simulink model "stereo_ibvs_core_backup_20260724_004703"  (R2025b)
settings: Solver=FixedStepDiscrete  StartTime=0.0  StopTime=inf  FixedStep=cfg.Ts  RelTol=1e-3
InitFcn:
  | cfgValid__=evalin('base','exist(''cfg'',''var'')==1 && isstruct(cfg) && all(isfield(cfg,{''Ts'',''robot'',''qInitial'',''zoomInitialSteps'',''cameraIntrinsicsStage1'',''rhoD'',''stereoBaseline'',''centerDesired'',''Kc'',''lambdaC'',''qMin'',''qMax'',''qLimitSoftMargin'',''qDotAlgorithmMax'',''stage1CalibrationReady''}))');if ~cfgValid__,modelFile__=get_param(bdroot,'FileName');modelDir__=fileparts(modelFile__);config1__=fullfile(modelDir__,'stereo_ibvs_config.m');config2__=fullfile(fileparts(modelDir__),'config','stereo_ibvs_config.m');if isfile(config1__),run(config1__);elseif isfile(config2__),run(config2__);else,error('StereoIBVS:ConfigNotFound','找不到stereo_ibvs_config.m。');end;end;clear cfgValid__ modelFile__ modelDir__ config1__ config2__
undefined symbols (not defined in the file): cfg, cfg_baseline, cfg_ekfCovarianceJitter, cfg_ekfInitializationMode, cfg_ekfP0, cfg_ekfRequireNewMeasurement, cfg_ekfSConditionMin, cfg_ekfX0, cfg_focalLength0Mm, cfg_fr3Axis, cfg_fr3Joint8OriginRPY, cfg_fr3Joint8OriginXYZ, cfg_fr3OriginRPY, cfg_fr3OriginXYZ, cfg_numericalEpsilon, cfg_pixelNoiseStd, cfg_q0, cfg_rhoMax, cfg_rhoMin, cfg_sigmaJerk, cfg_T_CL_CR, cfg_T_link8_CL, cfg_T_W_B, cfg_Ts, cfg_visibilityZMin
(part 1 of 4)
settings Model: Creator=harry  LastModifiedBy=harry

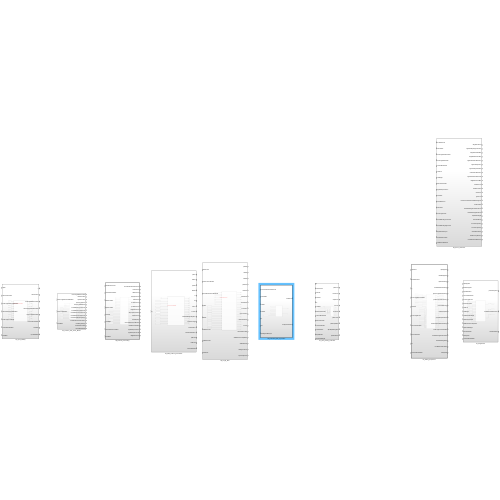
[thumbnail: Simulink's stored preview of the top-level diagram]
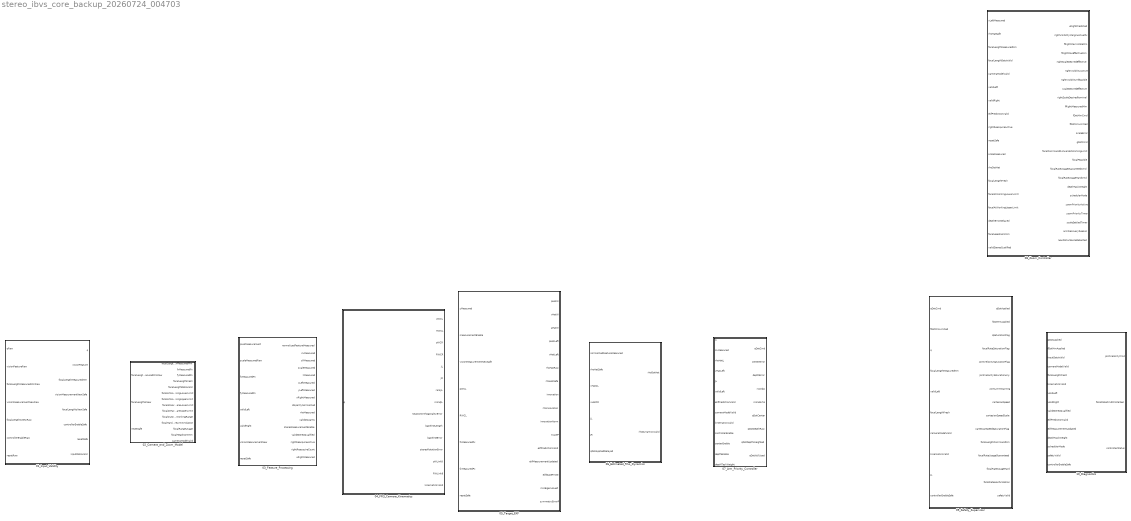
== system stereo_ibvs_core_backup_20260724_004703 ==
  01_Input_Validity : Subsystem
  02_Camera_and_Zoom_Model : Subsystem
  03_Feature_Processing : Subsystem  Description=将像素坐标转换为左右相机归一化坐标，并检查输入有效性。  TreatAsAtomicUnit=on
  04_FR3_Camera_Kinematics : Subsystem
  05_Target_EKF : Subsystem
  06_Estimated_Rho_Dynamics : Subsystem  TreatAsAtomicUnit=on
  07_Arm_Priority_Controller : Subsystem
  08_Zoom_Controller : Subsystem
  09_Safety_Supervisor : Subsystem  TreatAsAtomicUnit=on
  10_Diagnostics : Subsystem

== system stereo_ibvs_core_backup_20260724_004703/01_Input_Validity ==
  qRaw : Inport  OutDataTypeStr=double  PortDimensions=[7 1]
  visionFeatureRaw : Inport  Port=2  OutDataTypeStr=double  PortDimensions=[8 1]
  focalLengthMeasuredMmRaw : Inport  Port=3  OutDataTypeStr=double  PortDimensions=[2 1]
  visionMeasurementNewRaw : Inport  Port=4  OutDataTypeStr=double  PortDimensions=1
  focalLengthIsNewRaw : Inport  Port=5  OutDataTypeStr=double  PortDimensions=1
  controllerEnableRaw : Inport  Port=6  OutDataTypeStr=double  PortDimensions=1
  resetRaw : Inport  Port=7  OutDataTypeStr=double  PortDimensions=1
  Initial Focal Length Mm : Constant  Value=cfg_focalLength0Mm  OutDataTypeStr=double
  Initial Joint Position : Constant  Value=cfg_q0  OutDataTypeStr=double
  Input Validity : MATLAB Function  TreatAsAtomicUnit=on
  q : Outport  PortDimensions=[7 1]
  visionFeature : Outport  Port=2  PortDimensions=[8 1]
  focalLengthMeasuredMm : Outport  Port=3  PortDimensions=[2 1]
  visionMeasurementNewSafe : Outport  Port=4  PortDimensions=1
  focalLengthIsNewSafe : Outport  Port=5  PortDimensions=1
  controllerEnableSafe : Outport  Port=6  PortDimensions=1
  resetSafe : Outport  Port=7  PortDimensions=1
  inputDataValid : Outport  Port=8  PortDimensions=1
  wires:
  ? -> ?
  qRaw/1 -> Input Validity/1(qRaw)
  visionFeatureRaw/1 -> Input Validity/2(visionFeatureRaw)
  focalLengthMeasuredMmRaw/1 -> Input Validity/3(focalLengthMeasuredMmRaw)
  visionMeasurementNewRaw/1 -> Input Validity/4(visionMeasurementNewRaw)
  focalLengthIsNewRaw/1 -> Input Validity/5(focalLengthIsNewRaw)
  controllerEnableRaw/1 -> Input Validity/6(controllerEnableRaw)
  resetRaw/1 -> Input Validity/7(resetRaw)
  Initial Joint Position/1 -> Input Validity/8(qInitial)
  Initial Focal Length Mm/1 -> Input Validity/9(focalLength0Mm)
  Input Validity/1(q) -> q/1
  Input Validity/2(visionFeature) -> visionFeature/1
  Input Validity/3(focalLengthMeasuredMm) -> focalLengthMeasuredMm/1
  Input Validity/4(visionMeasurementNewSafe) -> visionMeasurementNewSafe/1
  Input Validity/5(focalLengthIsNewSafe) -> focalLengthIsNewSafe/1
  Input Validity/6(controllerEnableSafe) -> controllerEnableSafe/1
  Input Validity/7(resetSafe) -> resetSafe/1
  Input Validity/8(inputDataValid) -> inputDataValid/1

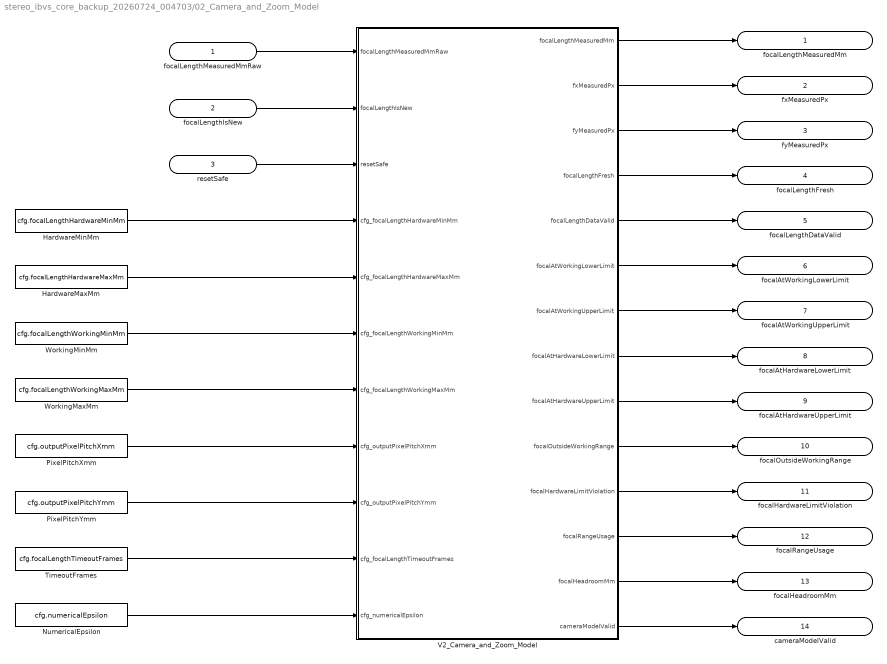
== system stereo_ibvs_core_backup_20260724_004703/02_Camera_and_Zoom_Model ==
  focalLengthMeasuredMmRaw : Inport  PortDimensions=2
  focalLengthIsNew : Inport  Port=2  PortDimensions=1
  resetSafe : Inport  Port=3  PortDimensions=1
  HardwareMaxMm : Constant  Value=cfg.focalLengthHardwareMaxMm
  HardwareMinMm : Constant  Value=cfg.focalLengthHardwareMinMm
  NumericalEpsilon : Constant  Value=cfg.numericalEpsilon
  PixelPitchXmm : Constant  Value=cfg.outputPixelPitchXmm
  PixelPitchYmm : Constant  Value=cfg.outputPixelPitchYmm
  TimeoutFrames : Constant  Value=cfg.focalLengthTimeoutFrames
  V2_Camera_and_Zoom_Model : MATLAB Function  TreatAsAtomicUnit=on
  WorkingMaxMm : Constant  Value=cfg.focalLengthWorkingMaxMm
  WorkingMinMm : Constant  Value=cfg.focalLengthWorkingMinMm
  focalLengthMeasuredMm : Outport  PortDimensions=2
  fxMeasuredPx : Outport  Port=2  PortDimensions=2
  fyMeasuredPx : Outport  Port=3  PortDimensions=2
  focalLengthFresh : Outport  Port=4  PortDimensions=1
  focalLengthDataValid : Outport  Port=5  PortDimensions=1
  focalAtWorkingLowerLimit : Outport  Port=6  PortDimensions=2
  focalAtWorkingUpperLimit : Outport  Port=7  PortDimensions=2
  focalAtHardwareLowerLimit : Outport  Port=8  PortDimensions=2
  focalAtHardwareUpperLimit : Outport  Port=9  PortDimensions=2
  focalOutsideWorkingRange : Outport  Port=10  PortDimensions=2
  focalHardwareLimitViolation : Outport  Port=11  PortDimensions=2
  focalRangeUsage : Outport  Port=12  PortDimensions=2
  focalHeadroomMm : Outport  Port=13  PortDimensions=2
  cameraModelValid : Outport  Port=14  PortDimensions=1
  wires:
  V2_Camera_and_Zoom_Model/13(focalHeadroomMm) -> focalHeadroomMm/1
  V2_Camera_and_Zoom_Model/12(focalRangeUsage) -> focalRangeUsage/1
  V2_Camera_and_Zoom_Model/11(focalHardwareLimitViolation) -> focalHardwareLimitViolation/1
  V2_Camera_and_Zoom_Model/10(focalOutsideWorkingRange) -> focalOutsideWorkingRange/1
  V2_Camera_and_Zoom_Model/14(cameraModelValid) -> cameraModelValid/1
  V2_Camera_and_Zoom_Model/9(focalAtHardwareUpperLimit) -> focalAtHardwareUpperLimit/1
  V2_Camera_and_Zoom_Model/6(focalAtWorkingLowerLimit) -> focalAtWorkingLowerLimit/1
  V2_Camera_and_Zoom_Model/4(focalLengthFresh) -> focalLengthFresh/1
  focalLengthMeasuredMmRaw/1 -> V2_Camera_and_Zoom_Model/1(focalLengthMeasuredMmRaw)
  focalLengthIsNew/1 -> V2_Camera_and_Zoom_Model/2(focalLengthIsNew)
  WorkingMinMm/1 -> V2_Camera_and_Zoom_Model/6(cfg_focalLengthWorkingMinMm)
  V2_Camera_and_Zoom_Model/3(fyMeasuredPx) -> fyMeasuredPx/1
  PixelPitchXmm/1 -> V2_Camera_and_Zoom_Model/8(cfg_outputPixelPitchXmm)
  V2_Camera_and_Zoom_Model/7(focalAtWorkingUpperLimit) -> focalAtWorkingUpperLimit/1
  TimeoutFrames/1 -> V2_Camera_and_Zoom_Model/10(cfg_focalLengthTimeoutFrames)
  V2_Camera_and_Zoom_Model/5(focalLengthDataValid) -> focalLengthDataValid/1
  resetSafe/1 -> V2_Camera_and_Zoom_Model/3(resetSafe)
  HardwareMinMm/1 -> V2_Camera_and_Zoom_Model/4(cfg_focalLengthHardwareMinMm)
  V2_Camera_and_Zoom_Model/8(focalAtHardwareLowerLimit) -> focalAtHardwareLowerLimit/1
  HardwareMaxMm/1 -> V2_Camera_and_Zoom_Model/5(cfg_focalLengthHardwareMaxMm)
  WorkingMaxMm/1 -> V2_Camera_and_Zoom_Model/7(cfg_focalLengthWorkingMaxMm)
  V2_Camera_and_Zoom_Model/1(focalLengthMeasuredMm) -> focalLengthMeasuredMm/1
  NumericalEpsilon/1 -> V2_Camera_and_Zoom_Model/11(cfg_numericalEpsilon)
  PixelPitchYmm/1 -> V2_Camera_and_Zoom_Model/9(cfg_outputPixelPitchYmm)
  V2_Camera_and_Zoom_Model/2(fxMeasuredPx) -> fxMeasuredPx/1

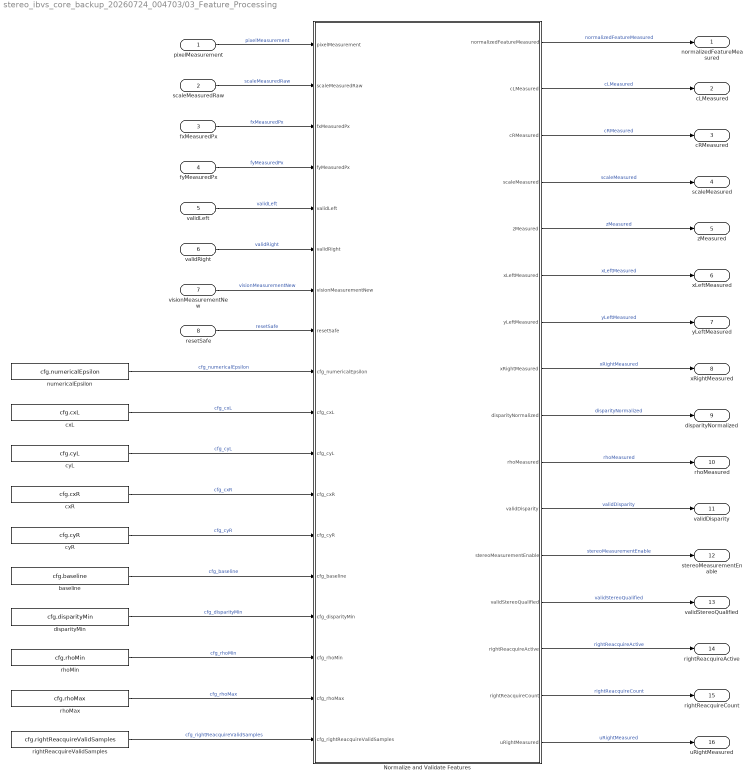
== system stereo_ibvs_core_backup_20260724_004703/03_Feature_Processing ==
  pixelMeasurement : Inport  OutDataTypeStr=double  PortDimensions=[4 1]
  scaleMeasuredRaw : Inport  Port=2  OutDataTypeStr=double  PortDimensions=[2 1]
  fxMeasuredPx : Inport  Port=3  OutDataTypeStr=double  PortDimensions=[2 1]
  fyMeasuredPx : Inport  Port=4  OutDataTypeStr=double  PortDimensions=[2 1]
  validLeft : Inport  Port=5  OutDataTypeStr=double  PortDimensions=1
  validRight : Inport  Port=6  OutDataTypeStr=double  PortDimensions=1
  visionMeasurementNew : Inport  Port=7  OutDataTypeStr=double  PortDimensions=1
  resetSafe : Inport  Port=8  OutDataTypeStr=double  PortDimensions=1
  Normalize and Validate Features : MATLAB Function  TreatAsAtomicUnit=on
  baseline : Constant  Value=cfg.baseline  OutDataTypeStr=double  SampleTime=-1
  cxL : Constant  Value=cfg.cxL  OutDataTypeStr=double  SampleTime=-1
  cxR : Constant  Value=cfg.cxR  OutDataTypeStr=double  SampleTime=-1
  cyL : Constant  Value=cfg.cyL  OutDataTypeStr=double  SampleTime=-1
  cyR : Constant  Value=cfg.cyR  OutDataTypeStr=double  SampleTime=-1
  disparityMin : Constant  Value=cfg.disparityMin  OutDataTypeStr=double  SampleTime=-1
  numericalEpsilon : Constant  Value=cfg.numericalEpsilon  OutDataTypeStr=double  SampleTime=-1
  rhoMax : Constant  Value=cfg.rhoMax  OutDataTypeStr=double  SampleTime=-1
  rhoMin : Constant  Value=cfg.rhoMin  OutDataTypeStr=double  SampleTime=-1
  rightReacquireValidSamples : Constant  Value=cfg.rightReacquireValidSamples  OutDataTypeStr=double  SampleTime=-1
  normalizedFeatureMeasured : Outport  PortDimensions=[4 1]
  cLMeasured : Outport  Port=2  PortDimensions=[2 1]
  cRMeasured : Outport  Port=3  PortDimensions=[2 1]
  scaleMeasured : Outport  Port=4  PortDimensions=[2 1]
  zMeasured : Outport  Port=5  PortDimensions=[3 1]
  xLeftMeasured : Outport  Port=6  PortDimensions=1
  yLeftMeasured : Outport  Port=7  PortDimensions=1
  xRightMeasured : Outport  Port=8  PortDimensions=1
  disparityNormalized : Outport  Port=9  PortDimensions=1
  rhoMeasured : Outport  Port=10  PortDimensions=1
  validDisparity : Outport  Port=11  PortDimensions=1
  stereoMeasurementEnable : Outport  Port=12  PortDimensions=1
  validStereoQualified : Outport  Port=13  PortDimensions=1
  rightReacquireActive : Outport  Port=14  PortDimensions=1
  rightReacquireCount : Outport  Port=15  PortDimensions=1
  uRightMeasured : Outport  Port=16  PortDimensions=1
  wires:
  pixelMeasurement/1 -> Normalize and Validate Features/1(pixelMeasurement)  "pixelMeasurement"
  scaleMeasuredRaw/1 -> Normalize and Validate Features/2(scaleMeasuredRaw)  "scaleMeasuredRaw"
  fxMeasuredPx/1 -> Normalize and Validate Features/3(fxMeasuredPx)  "fxMeasuredPx"
  fyMeasuredPx/1 -> Normalize and Validate Features/4(fyMeasuredPx)  "fyMeasuredPx"
  validLeft/1 -> Normalize and Validate Features/5(validLeft)  "validLeft"
  validRight/1 -> Normalize and Validate Features/6(validRight)  "validRight"
  visionMeasurementNew/1 -> Normalize and Validate Features/7(visionMeasurementNew)  "visionMeasurementNew"
  resetSafe/1 -> Normalize and Validate Features/8(resetSafe)  "resetSafe"
  numericalEpsilon/1 -> Normalize and Validate Features/9(cfg_numericalEpsilon)  "cfg_numericalEpsilon"
  cxL/1 -> Normalize and Validate Features/10(cfg_cxL)  "cfg_cxL"
  cyL/1 -> Normalize and Validate Features/11(cfg_cyL)  "cfg_cyL"
  cxR/1 -> Normalize and Validate Features/12(cfg_cxR)  "cfg_cxR"
  cyR/1 -> Normalize and Validate Features/13(cfg_cyR)  "cfg_cyR"
  baseline/1 -> Normalize and Validate Features/14(cfg_baseline)  "cfg_baseline"
  disparityMin/1 -> Normalize and Validate Features/15(cfg_disparityMin)  "cfg_disparityMin"
  rhoMin/1 -> Normalize and Validate Features/16(cfg_rhoMin)  "cfg_rhoMin"
  rhoMax/1 -> Normalize and Validate Features/17(cfg_rhoMax)  "cfg_rhoMax"
  rightReacquireValidSamples/1 -> Normalize and Validate Features/18(cfg_rightReacquireValidSamples)  "cfg_rightReacquireValidSamples"
  Normalize and Validate Features/1(normalizedFeatureMeasured) -> normalizedFeatureMeasured/1  "normalizedFeatureMeasured"
  Normalize and Validate Features/2(cLMeasured) -> cLMeasured/1  "cLMeasured"
  Normalize and Validate Features/3(cRMeasured) -> cRMeasured/1  "cRMeasured"
  Normalize and Validate Features/4(scaleMeasured) -> scaleMeasured/1  "scaleMeasured"
  Normalize and Validate Features/5(zMeasured) -> zMeasured/1  "zMeasured"
  Normalize and Validate Features/6(xLeftMeasured) -> xLeftMeasured/1  "xLeftMeasured"
  Normalize and Validate Features/7(yLeftMeasured) -> yLeftMeasured/1  "yLeftMeasured"
  Normalize and Validate Features/8(xRightMeasured) -> xRightMeasured/1  "xRightMeasured"
  Normalize and Validate Features/9(disparityNormalized) -> disparityNormalized/1  "disparityNormalized"
  Normalize and Validate Features/10(rhoMeasured) -> rhoMeasured/1  "rhoMeasured"
  Normalize and Validate Features/11(validDisparity) -> validDisparity/1  "validDisparity"
  Normalize and Validate Features/12(stereoMeasurementEnable) -> stereoMeasurementEnable/1  "stereoMeasurementEnable"
  Normalize and Validate Features/13(validStereoQualified) -> validStereoQualified/1  "validStereoQualified"
  Normalize and Validate Features/14(rightReacquireActive) -> rightReacquireActive/1  "rightReacquireActive"
  Normalize and Validate Features/15(rightReacquireCount) -> rightReacquireCount/1  "rightReacquireCount"
  Normalize and Validate Features/16(uRightMeasured) -> uRightMeasured/1  "uRightMeasured"

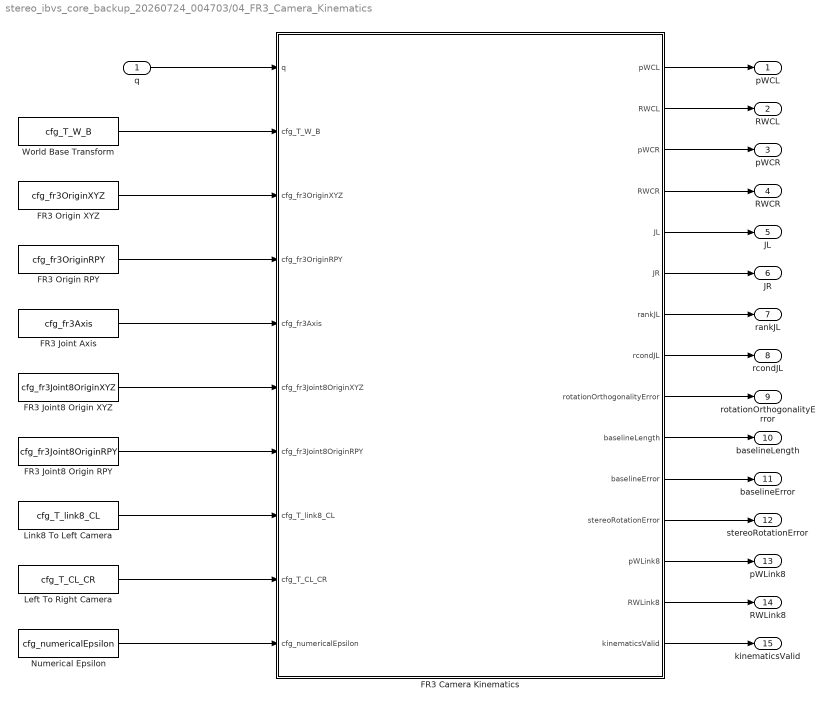
== system stereo_ibvs_core_backup_20260724_004703/04_FR3_Camera_Kinematics ==
  q : Inport  OutDataTypeStr=double  PortDimensions=[7 1]
  FR3 Camera Kinematics : MATLAB Function  TreatAsAtomicUnit=on
  FR3 Joint Axis : Constant  Value=cfg_fr3Axis  OutDataTypeStr=double  SampleTime=-1
  FR3 Joint8 Origin RPY : Constant  Value=cfg_fr3Joint8OriginRPY  OutDataTypeStr=double  SampleTime=-1
  FR3 Joint8 Origin XYZ : Constant  Value=cfg_fr3Joint8OriginXYZ  OutDataTypeStr=double  SampleTime=-1
  FR3 Origin RPY : Constant  Value=cfg_fr3OriginRPY  OutDataTypeStr=double  SampleTime=-1
  FR3 Origin XYZ : Constant  Value=cfg_fr3OriginXYZ  OutDataTypeStr=double  SampleTime=-1
  Left To Right Camera : Constant  Value=cfg_T_CL_CR  OutDataTypeStr=double  SampleTime=-1
  Link8 To Left Camera : Constant  Value=cfg_T_link8_CL  OutDataTypeStr=double  SampleTime=-1
  Numerical Epsilon : Constant  Value=cfg_numericalEpsilon  OutDataTypeStr=double  SampleTime=-1
  World Base Transform : Constant  Value=cfg_T_W_B  OutDataTypeStr=double  SampleTime=-1
  pWCL : Outport  PortDimensions=[3 1]
  RWCL : Outport  Port=2  PortDimensions=[3 3]
  pWCR : Outport  Port=3  PortDimensions=[3 1]
  RWCR : Outport  Port=4  PortDimensions=[3 3]
  JL : Outport  Port=5  PortDimensions=[6 7]
  JR : Outport  Port=6  PortDimensions=[6 7]
  rankJL : Outport  Port=7  PortDimensions=1
  rcondJL : Outport  Port=8  PortDimensions=1
  rotationOrthogonalityError : Outport  Port=9  PortDimensions=1
  baselineLength : Outport  Port=10  PortDimensions=1
  baselineError : Outport  Port=11  PortDimensions=1
  stereoRotationError : Outport  Port=12  PortDimensions=1
  pWLink8 : Outport  Port=13  PortDimensions=[3 1]
  RWLink8 : Outport  Port=14  PortDimensions=[3 3]
  kinematicsValid : Outport  Port=15  PortDimensions=1
  wires:
  ? -> ?
  q/1 -> FR3 Camera Kinematics/1(q)
  World Base Transform/1 -> FR3 Camera Kinematics/2(cfg_T_W_B)
  FR3 Origin XYZ/1 -> FR3 Camera Kinematics/3(cfg_fr3OriginXYZ)
  FR3 Origin RPY/1 -> FR3 Camera Kinematics/4(cfg_fr3OriginRPY)
  FR3 Joint Axis/1 -> FR3 Camera Kinematics/5(cfg_fr3Axis)
  FR3 Joint8 Origin XYZ/1 -> FR3 Camera Kinematics/6(cfg_fr3Joint8OriginXYZ)
  FR3 Joint8 Origin RPY/1 -> FR3 Camera Kinematics/7(cfg_fr3Joint8OriginRPY)
  Link8 To Left Camera/1 -> FR3 Camera Kinematics/8(cfg_T_link8_CL)
  Left To Right Camera/1 -> FR3 Camera Kinematics/9(cfg_T_CL_CR)
  Numerical Epsilon/1 -> FR3 Camera Kinematics/10(cfg_numericalEpsilon)
  FR3 Camera Kinematics/1(pWCL) -> pWCL/1
  FR3 Camera Kinematics/2(RWCL) -> RWCL/1
  FR3 Camera Kinematics/3(pWCR) -> pWCR/1
  FR3 Camera Kinematics/4(RWCR) -> RWCR/1
  FR3 Camera Kinematics/5(JL) -> JL/1
  FR3 Camera Kinematics/6(JR) -> JR/1
  FR3 Camera Kinematics/7(rankJL) -> rankJL/1
  FR3 Camera Kinematics/8(rcondJL) -> rcondJL/1
  FR3 Camera Kinematics/9(rotationOrthogonalityError) -> rotationOrthogonalityError/1
  FR3 Camera Kinematics/10(baselineLength) -> baselineLength/1
  FR3 Camera Kinematics/11(baselineError) -> baselineError/1
  FR3 Camera Kinematics/12(stereoRotationError) -> stereoRotationError/1
  FR3 Camera Kinematics/13(pWLink8) -> pWLink8/1
  FR3 Camera Kinematics/14(RWLink8) -> RWLink8/1
  FR3 Camera Kinematics/15(kinematicsValid) -> kinematicsValid/1

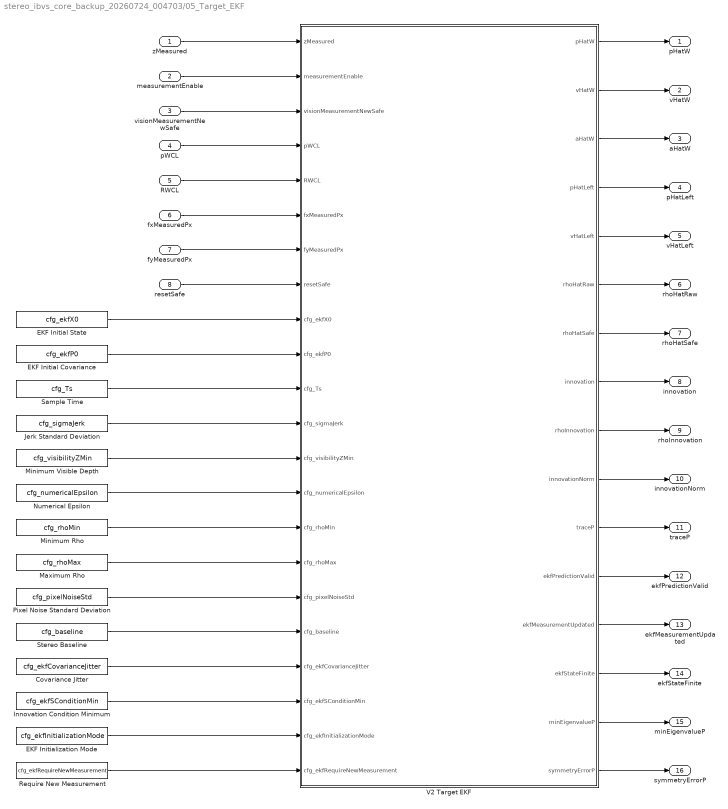
== system stereo_ibvs_core_backup_20260724_004703/05_Target_EKF ==
  zMeasured : Inport  OutDataTypeStr=double  PortDimensions=[3 1]
  measurementEnable : Inport  Port=2  OutDataTypeStr=double  PortDimensions=1
  visionMeasurementNewSafe : Inport  Port=3  OutDataTypeStr=double  PortDimensions=1
  pWCL : Inport  Port=4  OutDataTypeStr=double  PortDimensions=[3 1]
  RWCL : Inport  Port=5  OutDataTypeStr=double  PortDimensions=[3 3]
  fxMeasuredPx : Inport  Port=6  OutDataTypeStr=double  PortDimensions=[2 1]
  fyMeasuredPx : Inport  Port=7  OutDataTypeStr=double  PortDimensions=[2 1]
  resetSafe : Inport  Port=8  OutDataTypeStr=double  PortDimensions=1
  Covariance Jitter : Constant  Value=cfg_ekfCovarianceJitter  OutDataTypeStr=double  SampleTime=-1
  EKF Initial Covariance : Constant  Value=cfg_ekfP0  OutDataTypeStr=double  SampleTime=-1
  EKF Initial State : Constant  Value=cfg_ekfX0  OutDataTypeStr=double  SampleTime=-1
  EKF Initialization Mode : Constant  Value=cfg_ekfInitializationMode  OutDataTypeStr=double  SampleTime=-1
  Innovation Condition Minimum : Constant  Value=cfg_ekfSConditionMin  OutDataTypeStr=double  SampleTime=-1
  Jerk Standard Deviation : Constant  Value=cfg_sigmaJerk  OutDataTypeStr=double  SampleTime=-1
  Maximum Rho : Constant  Value=cfg_rhoMax  OutDataTypeStr=double  SampleTime=-1
  Minimum Rho : Constant  Value=cfg_rhoMin  OutDataTypeStr=double  SampleTime=-1
  Minimum Visible Depth : Constant  Value=cfg_visibilityZMin  OutDataTypeStr=double  SampleTime=-1
  Numerical Epsilon : Constant  Value=cfg_numericalEpsilon  OutDataTypeStr=double  SampleTime=-1
  Pixel Noise Standard Deviation : Constant  Value=cfg_pixelNoiseStd  OutDataTypeStr=double  SampleTime=-1
  Require New Measurement : Constant  Value=cfg_ekfRequireNewMeasurement  OutDataTypeStr=double  SampleTime=-1
  Sample Time : Constant  Value=cfg_Ts  OutDataTypeStr=double  SampleTime=-1
  Stereo Baseline : Constant  Value=cfg_baseline  OutDataTypeStr=double  SampleTime=-1
  V2 Target EKF : MATLAB Function  TreatAsAtomicUnit=on
  pHatW : Outport  PortDimensions=[3 1]
  vHatW : Outport  Port=2  PortDimensions=[3 1]
  aHatW : Outport  Port=3  PortDimensions=[3 1]
  pHatLeft : Outport  Port=4  PortDimensions=[3 1]
  vHatLeft : Outport  Port=5  PortDimensions=[3 1]
  rhoHatRaw : Outport  Port=6  PortDimensions=1
  rhoHatSafe : Outport  Port=7  PortDimensions=1
  innovation : Outport  Port=8  PortDimensions=[3 1]
  rhoInnovation : Outport  Port=9  PortDimensions=1
  innovationNorm : Outport  Port=10  PortDimensions=1
  traceP : Outport  Port=11  PortDimensions=1
  ekfPredictionValid : Outport  Port=12  PortDimensions=1
  ekfMeasurementUpdated : Outport  Port=13  PortDimensions=1
  ekfStateFinite : Outport  Port=14  PortDimensions=1
  minEigenvalueP : Outport  Port=15  PortDimensions=1
  symmetryErrorP : Outport  Port=16  PortDimensions=1
  wires:
  ? -> ?
  zMeasured/1 -> V2 Target EKF/1(zMeasured)
  measurementEnable/1 -> V2 Target EKF/2(measurementEnable)
  visionMeasurementNewSafe/1 -> V2 Target EKF/3(visionMeasurementNewSafe)
  pWCL/1 -> V2 Target EKF/4(pWCL)
  RWCL/1 -> V2 Target EKF/5(RWCL)
  fxMeasuredPx/1 -> V2 Target EKF/6(fxMeasuredPx)
  fyMeasuredPx/1 -> V2 Target EKF/7(fyMeasuredPx)
  resetSafe/1 -> V2 Target EKF/8(resetSafe)
  EKF Initial State/1 -> V2 Target EKF/9(cfg_ekfX0)
  EKF Initial Covariance/1 -> V2 Target EKF/10(cfg_ekfP0)
  Sample Time/1 -> V2 Target EKF/11(cfg_Ts)
  Jerk Standard Deviation/1 -> V2 Target EKF/12(cfg_sigmaJerk)
  Minimum Visible Depth/1 -> V2 Target EKF/13(cfg_visibilityZMin)
  Numerical Epsilon/1 -> V2 Target EKF/14(cfg_numericalEpsilon)
  Minimum Rho/1 -> V2 Target EKF/15(cfg_rhoMin)
  Maximum Rho/1 -> V2 Target EKF/16(cfg_rhoMax)
  Pixel Noise Standard Deviation/1 -> V2 Target EKF/17(cfg_pixelNoiseStd)
  Stereo Baseline/1 -> V2 Target EKF/18(cfg_baseline)
  Covariance Jitter/1 -> V2 Target EKF/19(cfg_ekfCovarianceJitter)
  Innovation Condition Minimum/1 -> V2 Target EKF/20(cfg_ekfSConditionMin)
  EKF Initialization Mode/1 -> V2 Target EKF/21(cfg_ekfInitializationMode)
  Require New Measurement/1 -> V2 Target EKF/22(cfg_ekfRequireNewMeasurement)
  V2 Target EKF/1(pHatW) -> pHatW/1
  V2 Target EKF/2(vHatW) -> vHatW/1
  V2 Target EKF/3(aHatW) -> aHatW/1
  V2 Target EKF/4(pHatLeft) -> pHatLeft/1
  V2 Target EKF/5(vHatLeft) -> vHatLeft/1
  V2 Target EKF/6(rhoHatRaw) -> rhoHatRaw/1
  V2 Target EKF/7(rhoHatSafe) -> rhoHatSafe/1
  V2 Target EKF/8(innovation) -> innovation/1
  V2 Target EKF/9(rhoInnovation) -> rhoInnovation/1
  V2 Target EKF/10(innovationNorm) -> innovationNorm/1
  V2 Target EKF/11(traceP) -> traceP/1
  V2 Target EKF/12(ekfPredictionValid) -> ekfPredictionValid/1
  V2 Target EKF/13(ekfMeasurementUpdated) -> ekfMeasurementUpdated/1
  V2 Target EKF/14(ekfStateFinite) -> ekfStateFinite/1
  V2 Target EKF/15(minEigenvalueP) -> minEigenvalueP/1
  V2 Target EKF/16(symmetryErrorP) -> symmetryErrorP/1

== system stereo_ibvs_core_backup_20260724_004703/06_Estimated_Rho_Dynamics ==
  normalizedFeatureMeasured : Inport  OutDataTypeStr=double  PortDimensions=[4 1]
  rhoHatSafe : Inport  Port=2  OutDataTypeStr=double  PortDimensions=1
  vHatCL : Inport  Port=3  OutDataTypeStr=double  PortDimensions=[3 1]
  vHatCR : Inport  Port=4  OutDataTypeStr=double  PortDimensions=[3 1]
  JL : Inport  Port=5  OutDataTypeStr=double  PortDimensions=[6 7]
  JR : Inport  Port=6  OutDataTypeStr=double  PortDimensions=[6 7]
  qDotAppliedDelayed : Inport  Port=7  OutDataTypeStr=double  PortDimensions=[7 1]
  Estimate Rho Dynamics : MATLAB Function  TreatAsAtomicUnit=on
  numericalEpsilon : Constant  Value=cfg.numericalEpsilon  OutDataTypeStr=double  SampleTime=-1
  rhoDotHat : Outport  PortDimensions=[2 1]
  rhoDynamicsValid : Outport  Port=2  PortDimensions=1
  wires:
  normalizedFeatureMeasured/1 -> Estimate Rho Dynamics/1(normalizedFeatureMeasured)  "normalizedFeatureMeasured"
  rhoHatSafe/1 -> Estimate Rho Dynamics/2(rhoHatSafe)  "rhoHatSafe"
  vHatCL/1 -> Estimate Rho Dynamics/3(vHatCL)  "vHatCL"
  vHatCR/1 -> Estimate Rho Dynamics/4(vHatCR)  "vHatCR"
  JL/1 -> Estimate Rho Dynamics/5(JL)  "JL"
  JR/1 -> Estimate Rho Dynamics/6(JR)  "JR"
  qDotAppliedDelayed/1 -> Estimate Rho Dynamics/7(qDotAppliedDelayed)  "qDotAppliedDelayed"
  numericalEpsilon/1 -> Estimate Rho Dynamics/8(cfg_numericalEpsilon)  "cfg_numericalEpsilon"
  Estimate Rho Dynamics/1(rhoDotHat) -> rhoDotHat/1  "rhoDotHat"
  Estimate Rho Dynamics/2(rhoDynamicsValid) -> rhoDynamicsValid/1  "rhoDynamicsValid"

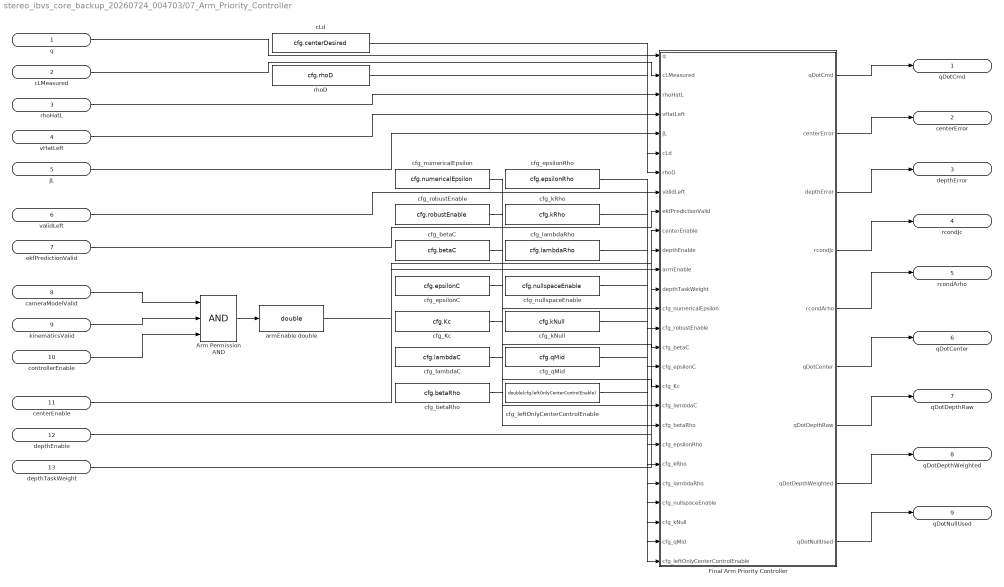
== system stereo_ibvs_core_backup_20260724_004703/07_Arm_Priority_Controller ==
  q : Inport
  cLMeasured : Inport  Port=2
  rhoHatL : Inport  Port=3
  vHatLeft : Inport  Port=4
  JL : Inport  Port=5
  validLeft : Inport  Port=6
  ekfPredictionValid : Inport  Port=7
  cameraModelValid : Inport  Port=8
  kinematicsValid : Inport  Port=9
  controllerEnable : Inport  Port=10
  centerEnable : Inport  Port=11
  depthEnable : Inport  Port=12
  depthTaskWeight : Inport  Port=13
  Arm Permission AND : Logic  Inputs=3  AllPortsSameDT=off  OutDataTypeStr=boolean
  Final Arm Priority Controller : MATLAB Function  TreatAsAtomicUnit=on
  armEnable double : DataTypeConversion  OutDataTypeStr=double  SaturateOnIntegerOverflow=off  RndMeth=Floor
  cLd : Constant  Value=cfg.centerDesired  OutDataTypeStr=double
  cfg_Kc : Constant  Value=cfg.Kc  OutDataTypeStr=double
  cfg_betaC : Constant  Value=cfg.betaC  OutDataTypeStr=double
  cfg_betaRho : Constant  Value=cfg.betaRho  OutDataTypeStr=double
  cfg_epsilonC : Constant  Value=cfg.epsilonC  OutDataTypeStr=double
  cfg_epsilonRho : Constant  Value=cfg.epsilonRho  OutDataTypeStr=double
  cfg_kNull : Constant  Value=cfg.kNull  OutDataTypeStr=double
  cfg_kRho : Constant  Value=cfg.kRho  OutDataTypeStr=double
  cfg_lambdaC : Constant  Value=cfg.lambdaC  OutDataTypeStr=double
  cfg_lambdaRho : Constant  Value=cfg.lambdaRho  OutDataTypeStr=double
  cfg_leftOnlyCenterControlEnable : Constant  Value=double(cfg.leftOnlyCenterControlEnable)  OutDataTypeStr=double
  cfg_nullspaceEnable : Constant  Value=cfg.nullspaceEnable  OutDataTypeStr=double
  cfg_numericalEpsilon : Constant  Value=cfg.numericalEpsilon  OutDataTypeStr=double
  cfg_qMid : Constant  Value=cfg.qMid  OutDataTypeStr=double
  cfg_robustEnable : Constant  Value=cfg.robustEnable  OutDataTypeStr=double
  rhoD : Constant  Value=cfg.rhoD  OutDataTypeStr=double
  qDotCmd : Outport
  centerError : Outport  Port=2
  depthError : Outport  Port=3
  rcondJc : Outport  Port=4
  rcondArho : Outport  Port=5
  qDotCenter : Outport  Port=6
  qDotDepthRaw : Outport  Port=7
  qDotDepthWeighted : Outport  Port=8
  qDotNullUsed : Outport  Port=9
  wires:
  cameraModelValid/1 -> Arm Permission AND/1
  kinematicsValid/1 -> Arm Permission AND/2
  controllerEnable/1 -> Arm Permission AND/3
  Arm Permission AND/1 -> armEnable double/1
  q/1 -> Final Arm Priority Controller/1(q)
  cLMeasured/1 -> Final Arm Priority Controller/2(cLMeasured)
  rhoHatL/1 -> Final Arm Priority Controller/3(rhoHatL)
  vHatLeft/1 -> Final Arm Priority Controller/4(vHatLeft)
  JL/1 -> Final Arm Priority Controller/5(JL)
  cLd/1 -> Final Arm Priority Controller/6(cLd)
  rhoD/1 -> Final Arm Priority Controller/7(rhoD)
  validLeft/1 -> Final Arm Priority Controller/8(validLeft)
  ekfPredictionValid/1 -> Final Arm Priority Controller/9(ekfPredictionValid)
  centerEnable/1 -> Final Arm Priority Controller/10(centerEnable)
  depthEnable/1 -> Final Arm Priority Controller/11(depthEnable)
  armEnable double/1 -> Final Arm Priority Controller/12(armEnable)
  depthTaskWeight/1 -> Final Arm Priority Controller/13(depthTaskWeight)
  cfg_numericalEpsilon/1 -> Final Arm Priority Controller/14(cfg_numericalEpsilon)
  cfg_robustEnable/1 -> Final Arm Priority Controller/15(cfg_robustEnable)
  cfg_betaC/1 -> Final Arm Priority Controller/16(cfg_betaC)
  cfg_epsilonC/1 -> Final Arm Priority Controller/17(cfg_epsilonC)
  cfg_Kc/1 -> Final Arm Priority Controller/18(cfg_Kc)
  cfg_lambdaC/1 -> Final Arm Priority Controller/19(cfg_lambdaC)
  cfg_betaRho/1 -> Final Arm Priority Controller/20(cfg_betaRho)
  cfg_epsilonRho/1 -> Final Arm Priority Controller/21(cfg_epsilonRho)
  cfg_kRho/1 -> Final Arm Priority Controller/22(cfg_kRho)
  cfg_lambdaRho/1 -> Final Arm Priority Controller/23(cfg_lambdaRho)
  cfg_nullspaceEnable/1 -> Final Arm Priority Controller/24(cfg_nullspaceEnable)
  cfg_kNull/1 -> Final Arm Priority Controller/25(cfg_kNull)
  cfg_qMid/1 -> Final Arm Priority Controller/26(cfg_qMid)
  cfg_leftOnlyCenterControlEnable/1 -> Final Arm Priority Controller/27(cfg_leftOnlyCenterControlEnable)
  Final Arm Priority Controller/1(qDotCmd) -> qDotCmd/1
  Final Arm Priority Controller/2(centerError) -> centerError/1
  Final Arm Priority Controller/3(depthError) -> depthError/1
  Final Arm Priority Controller/4(rcondJc) -> rcondJc/1
  Final Arm Priority Controller/5(rcondArho) -> rcondArho/1
  Final Arm Priority Controller/6(qDotCenter) -> qDotCenter/1
  Final Arm Priority Controller/7(qDotDepthRaw) -> qDotDepthRaw/1
  Final Arm Priority Controller/8(qDotDepthWeighted) -> qDotDepthWeighted/1
  Final Arm Priority Controller/9(qDotNullUsed) -> qDotNullUsed/1

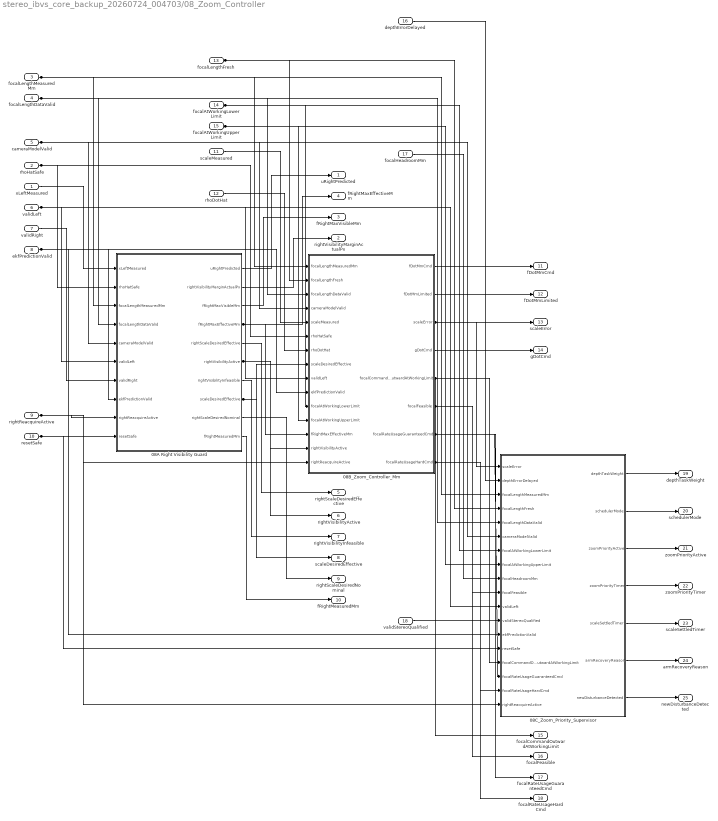
== system stereo_ibvs_core_backup_20260724_004703/08_Zoom_Controller ==
  xLeftMeasured : Inport  OutDataTypeStr=double  PortDimensions=1
  rhoHatSafe : Inport  Port=2  OutDataTypeStr=double  PortDimensions=1
  focalLengthMeasuredMm : Inport  Port=3  OutDataTypeStr=double  PortDimensions=[2 1]
  focalLengthDataValid : Inport  Port=4  OutDataTypeStr=double  PortDimensions=1
  cameraModelValid : Inport  Port=5  OutDataTypeStr=double  PortDimensions=1
  validLeft : Inport  Port=6  OutDataTypeStr=double  PortDimensions=1
  validRight : Inport  Port=7  OutDataTypeStr=double  PortDimensions=1
  ekfPredictionValid : Inport  Port=8  OutDataTypeStr=double  PortDimensions=1
  rightReacquireActive : Inport  Port=9  OutDataTypeStr=double  PortDimensions=1
  resetSafe : Inport  Port=10  OutDataTypeStr=double  PortDimensions=1
  scaleMeasured : Inport  Port=11  OutDataTypeStr=double  PortDimensions=[2 1]
  rhoDotHat : Inport  Port=12  OutDataTypeStr=double  PortDimensions=[2 1]
  focalLengthFresh : Inport  Port=13  OutDataTypeStr=double  PortDimensions=1
  focalAtWorkingLowerLimit : Inport  Port=14  OutDataTypeStr=double  PortDimensions=[2 1]
  focalAtWorkingUpperLimit : Inport  Port=15  OutDataTypeStr=double  PortDimensions=[2 1]
  depthErrorDelayed : Inport  Port=16  OutDataTypeStr=double  PortDimensions=1
  focalHeadroomMm : Inport  Port=17  OutDataTypeStr=double  PortDimensions=[2 1]
  validStereoQualified : Inport  Port=18  OutDataTypeStr=double  PortDimensions=1
  08A Right Visibility Guard : Subsystem
  08B_Zoom_Controller_Mm : Subsystem
  08C_Zoom_Priority_Supervisor : Subsystem
  uRightPredicted : Outport  PortDimensions=1
  rightVisibilityMarginActualPx : Outport  Port=2  PortDimensions=1
  fRightMaxVisibleMm : Outport  Port=3  PortDimensions=1
  fRightMaxEffectiveMm : Outport  Port=4  PortDimensions=1
  rightScaleDesiredEffective : Outport  Port=5  PortDimensions=1
  rightVisibilityActive : Outport  Port=6  PortDimensions=1
  rightVisibilityInfeasible : Outport  Port=7  PortDimensions=1
  scaleDesiredEffective : Outport  Port=8  PortDimensions=[2 1]
  rightScaleDesiredNominal : Outport  Port=9  PortDimensions=1
  fRightMeasuredMm : Outport  Port=10  PortDimensions=1
  fDotMmCmd : Outport  Port=11  PortDimensions=[2 1]
  fDotMmLimited : Outport  Port=12  PortDimensions=[2 1]
  scaleError : Outport  Port=13  PortDimensions=[2 1]
  gDotCmd : Outport  Port=14  PortDimensions=[2 1]
  focalCommandOutwardAtWorkingLimit : Outport  Port=15  PortDimensions=[2 1]
  focalFeasible : Outport  Port=16  PortDimensions=[2 1]
  focalRateUsageGuaranteedCmd : Outport  Port=17  PortDimensions=[2 1]
  focalRateUsageHardCmd : Outport  Port=18  PortDimensions=[2 1]
  depthTaskWeight : Outport  Port=19  PortDimensions=1
  schedulerMode : Outport  Port=20  PortDimensions=1
  zoomPriorityActive : Outport  Port=21  PortDimensions=1
  zoomPriorityTimer : Outport  Port=22  PortDimensions=1
  scaleSettledTimer : Outport  Port=23  PortDimensions=1
  armRecoveryReason : Outport  Port=24  PortDimensions=1
  newDisturbanceDetected : Outport  Port=25  PortDimensions=1
  wires:
  08C_Zoom_Priority_Supervisor/6(armRecoveryReason) -> armRecoveryReason/1
  08C_Zoom_Priority_Supervisor/5(scaleSettledTimer) -> scaleSettledTimer/1
  08C_Zoom_Priority_Supervisor/4(zoomPriorityTimer) -> zoomPriorityTimer/1
  08C_Zoom_Priority_Supervisor/2(schedulerMode) -> schedulerMode/1
  08C_Zoom_Priority_Supervisor/1(depthTaskWeight) -> depthTaskWeight/1
  08B_Zoom_Controller_Mm/8(focalRateUsageHardCmd) -> focalRateUsageHardCmd/1, 08C_Zoom_Priority_Supervisor/17(focalRateUsageHardCmd)
  08B_Zoom_Controller_Mm/5(focalCommandOutwardAtWorkingLimit) -> focalCommandOutwardAtWorkingLimit/1, 08C_Zoom_Priority_Supervisor/15(focalCommandOutwardAtWorkingLimit)
  08C_Zoom_Priority_Supervisor/7(newDisturbanceDetected) -> newDisturbanceDetected/1
  08B_Zoom_Controller_Mm/4(gDotCmd) -> gDotCmd/1
  08B_Zoom_Controller_Mm/3(scaleError) -> scaleError/1, 08C_Zoom_Priority_Supervisor/1(scaleError)
  focalAtWorkingLowerLimit/1 -> 08B_Zoom_Controller_Mm/11(focalAtWorkingLowerLimit), 08C_Zoom_Priority_Supervisor/7(focalAtWorkingLowerLimit)
  ekfPredictionValid/1 -> 08A Right Visibility Guard/8(ekfPredictionValid), 08B_Zoom_Controller_Mm/10(ekfPredictionValid), 08C_Zoom_Priority_Supervisor/13(ekfPredictionValid)
  08A Right Visibility Guard/7(rightVisibilityInfeasible) -> rightVisibilityInfeasible/1
  validRight/1 -> 08A Right Visibility Guard/7(validRight)
  validStereoQualified/1 -> 08C_Zoom_Priority_Supervisor/12(validStereoQualified)
  depthErrorDelayed/1 -> 08C_Zoom_Priority_Supervisor/2(depthErrorDelayed)
  08A Right Visibility Guard/3(fRightMaxVisibleMm) -> fRightMaxVisibleMm/1
  rightReacquireActive/1 -> 08A Right Visibility Guard/9(rightReacquireActive), 08B_Zoom_Controller_Mm/15(rightReacquireActive), 08C_Zoom_Priority_Supervisor/18(rightReacquireActive)
  rhoHatSafe/1 -> 08A Right Visibility Guard/2(rhoHatSafe), 08B_Zoom_Controller_Mm/6(rhoHatSafe)
  resetSafe/1 -> 08A Right Visibility Guard/10(resetSafe), 08C_Zoom_Priority_Supervisor/14(resetSafe)
  validLeft/1 -> 08A Right Visibility Guard/6(validLeft), 08C_Zoom_Priority_Supervisor/11(validLeft), 08B_Zoom_Controller_Mm/9(validLeft)
  cameraModelValid/1 -> 08A Right Visibility Guard/5(cameraModelValid), 08B_Zoom_Controller_Mm/4(cameraModelValid), 08C_Zoom_Priority_Supervisor/6(cameraModelValid)
  focalLengthDataValid/1 -> 08A Right Visibility Guard/4(focalLengthDataValid), 08B_Zoom_Controller_Mm/3(focalLengthDataValid), 08C_Zoom_Priority_Supervisor/5(focalLengthDataValid)
  08A Right Visibility Guard/1(uRightPredicted) -> uRightPredicted/1
  focalLengthFresh/1 -> 08B_Zoom_Controller_Mm/2(focalLengthFresh), 08C_Zoom_Priority_Supervisor/4(focalLengthFresh)
  focalLengthMeasuredMm/1 -> 08A Right Visibility Guard/3(focalLengthMeasuredMm), 08B_Zoom_Controller_Mm/1(focalLengthMeasuredMm), 08C_Zoom_Priority_Supervisor/3(focalLengthMeasuredMm)
  08B_Zoom_Controller_Mm/6(focalFeasible) -> focalFeasible/1, 08C_Zoom_Priority_Supervisor/10(focalFeasible)
  scaleMeasured/1 -> 08B_Zoom_Controller_Mm/5(scaleMeasured)
  08A Right Visibility Guard/9(rightScaleDesiredNominal) -> rightScaleDesiredNominal/1
  rhoDotHat/1 -> 08B_Zoom_Controller_Mm/7(rhoDotHat)
  xLeftMeasured/1 -> 08A Right Visibility Guard/1(xLeftMeasured)
  08A Right Visibility Guard/2(rightVisibilityMarginActualPx) -> rightVisibilityMarginActualPx/1
  08B_Zoom_Controller_Mm/7(focalRateUsageGuaranteedCmd) -> focalRateUsageGuaranteedCmd/1, 08C_Zoom_Priority_Supervisor/16(focalRateUsageGuaranteedCmd)
  08A Right Visibility Guard/4(fRightMaxEffectiveMm) -> fRightMaxEffectiveMm/1, 08B_Zoom_Controller_Mm/13(fRightMaxEffectiveMm)
  08A Right Visibility Guard/8(scaleDesiredEffective) -> scaleDesiredEffective/1, 08B_Zoom_Controller_Mm/8(scaleDesiredEffective)
  focalAtWorkingUpperLimit/1 -> 08B_Zoom_Controller_Mm/12(focalAtWorkingUpperLimit), 08C_Zoom_Priority_Supervisor/8(focalAtWorkingUpperLimit)
  08A Right Visibility Guard/6(rightVisibilityActive) -> rightVisibilityActive/1, 08B_Zoom_Controller_Mm/14(rightVisibilityActive)
  focalHeadroomMm/1 -> 08C_Zoom_Priority_Supervisor/9(focalHeadroomMm)
  08A Right Visibility Guard/10(fRightMeasuredMm) -> fRightMeasuredMm/1
  08A Right Visibility Guard/5(rightScaleDesiredEffective) -> rightScaleDesiredEffective/1
  08B_Zoom_Controller_Mm/1(fDotMmCmd) -> fDotMmCmd/1
  08C_Zoom_Priority_Supervisor/3(zoomPriorityActive) -> zoomPriorityActive/1
  08B_Zoom_Controller_Mm/2(fDotMmLimited) -> fDotMmLimited/1

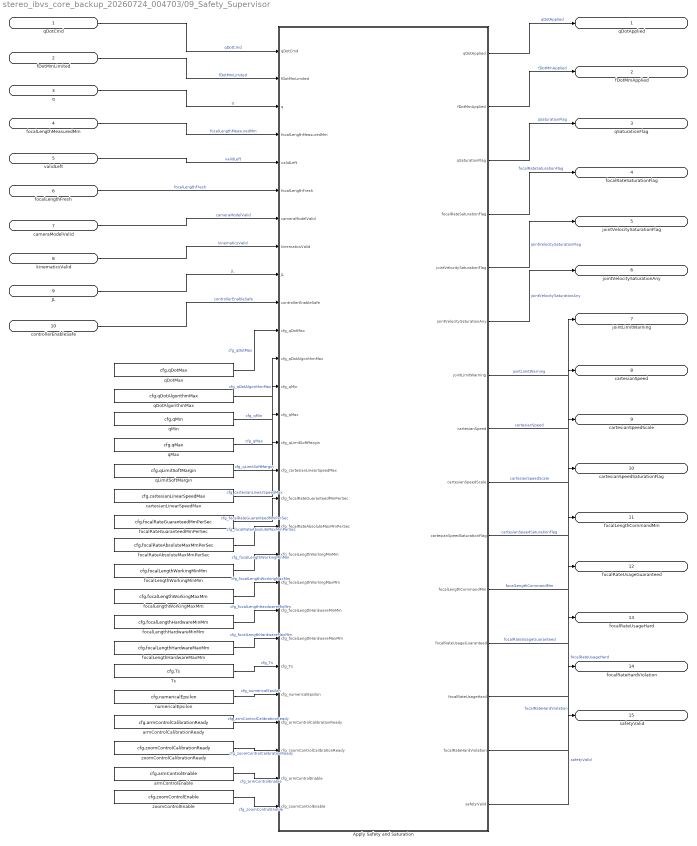
== system stereo_ibvs_core_backup_20260724_004703/09_Safety_Supervisor ==
  qDotCmd : Inport  OutDataTypeStr=double  PortDimensions=[7 1]
  fDotMmLimited : Inport  Port=2  OutDataTypeStr=double  PortDimensions=[2 1]
  q : Inport  Port=3  OutDataTypeStr=double  PortDimensions=[7 1]
  focalLengthMeasuredMm : Inport  Port=4  OutDataTypeStr=double  PortDimensions=[2 1]
  validLeft : Inport  Port=5  OutDataTypeStr=double  PortDimensions=1
  focalLengthFresh : Inport  Port=6  OutDataTypeStr=double  PortDimensions=1
  cameraModelValid : Inport  Port=7  OutDataTypeStr=double  PortDimensions=1
  kinematicsValid : Inport  Port=8  OutDataTypeStr=double  PortDimensions=1
  JL : Inport  Port=9  OutDataTypeStr=double  PortDimensions=[6 7]
  controllerEnableSafe : Inport  Port=10  OutDataTypeStr=double  PortDimensions=1
  Apply Safety and Saturation : MATLAB Function  TreatAsAtomicUnit=on
  Ts : Constant  Value=cfg.Ts  OutDataTypeStr=double  SampleTime=-1
  armControlCalibrationReady : Constant  Value=cfg.armControlCalibrationReady  OutDataTypeStr=double  SampleTime=-1
  armControlEnable : Constant  Value=cfg.armControlEnable  OutDataTypeStr=double  SampleTime=-1
  cartesianLinearSpeedMax : Constant  Value=cfg.cartesianLinearSpeedMax  OutDataTypeStr=double  SampleTime=-1
  focalLengthHardwareMaxMm : Constant  Value=cfg.focalLengthHardwareMaxMm  OutDataTypeStr=double  SampleTime=-1
  focalLengthHardwareMinMm : Constant  Value=cfg.focalLengthHardwareMinMm  OutDataTypeStr=double  SampleTime=-1
  focalLengthWorkingMaxMm : Constant  Value=cfg.focalLengthWorkingMaxMm  OutDataTypeStr=double  SampleTime=-1
  focalLengthWorkingMinMm : Constant  Value=cfg.focalLengthWorkingMinMm  OutDataTypeStr=double  SampleTime=-1
  focalRateAbsoluteMaxMmPerSec : Constant  Value=cfg.focalRateAbsoluteMaxMmPerSec  OutDataTypeStr=double  SampleTime=-1
  focalRateGuaranteedMmPerSec : Constant  Value=cfg.focalRateGuaranteedMmPerSec  OutDataTypeStr=double  SampleTime=-1
  numericalEpsilon : Constant  Value=cfg.numericalEpsilon  OutDataTypeStr=double  SampleTime=-1
  qDotAlgorithmMax : Constant  Value=cfg.qDotAlgorithmMax  OutDataTypeStr=double  SampleTime=-1
  qDotMax : Constant  Value=cfg.qDotMax  OutDataTypeStr=double  SampleTime=-1
  qLimitSoftMargin : Constant  Value=cfg.qLimitSoftMargin  OutDataTypeStr=double  SampleTime=-1
  qMax : Constant  Value=cfg.qMax  OutDataTypeStr=double  SampleTime=-1
  qMin : Constant  Value=cfg.qMin  OutDataTypeStr=double  SampleTime=-1
  zoomControlCalibrationReady : Constant  Value=cfg.zoomControlCalibrationReady  OutDataTypeStr=double  SampleTime=-1
  zoomControlEnable : Constant  Value=cfg.zoomControlEnable  OutDataTypeStr=double  SampleTime=-1
  qDotApplied : Outport  PortDimensions=[7 1]
  fDotMmApplied : Outport  Port=2  PortDimensions=[2 1]
  qSaturationFlag : Outport  Port=3  PortDimensions=1
  focalRateSaturationFlag : Outport  Port=4  PortDimensions=1
  jointVelocitySaturationFlag : Outport  Port=5  PortDimensions=[7 1]
  jointVelocitySaturationAny : Outport  Port=6  PortDimensions=1
  jointLimitWarning : Outport  Port=7  PortDimensions=[7 1]
  cartesianSpeed : Outport  Port=8  PortDimensions=1
  cartesianSpeedScale : Outport  Port=9  PortDimensions=1
  cartesianSpeedSaturationFlag : Outport  Port=10  PortDimensions=1
  focalLengthCommandMm : Outport  Port=11  PortDimensions=[2 1]
  focalRateUsageGuaranteed : Outport  Port=12  PortDimensions=[2 1]
  focalRateUsageHard : Outport  Port=13  PortDimensions=[2 1]
  focalRateHardViolation : Outport  Port=14  PortDimensions=[2 1]
  safetyValid : Outport  Port=15  PortDimensions=1
  wires:
  qDotCmd/1 -> Apply Safety and Saturation/1(qDotCmd)  "qDotCmd"
  fDotMmLimited/1 -> Apply Safety and Saturation/2(fDotMmLimited)  "fDotMmLimited"
  q/1 -> Apply Safety and Saturation/3(q)  "q"
  focalLengthMeasuredMm/1 -> Apply Safety and Saturation/4(focalLengthMeasuredMm)  "focalLengthMeasuredMm"
  validLeft/1 -> Apply Safety and Saturation/5(validLeft)  "validLeft"
  focalLengthFresh/1 -> Apply Safety and Saturation/6(focalLengthFresh)  "focalLengthFresh"
  cameraModelValid/1 -> Apply Safety and Saturation/7(cameraModelValid)  "cameraModelValid"
  kinematicsValid/1 -> Apply Safety and Saturation/8(kinematicsValid)  "kinematicsValid"
  JL/1 -> Apply Safety and Saturation/9(JL)  "JL"
  controllerEnableSafe/1 -> Apply Safety and Saturation/10(controllerEnableSafe)  "controllerEnableSafe"
  qDotMax/1 -> Apply Safety and Saturation/11(cfg_qDotMax)  "cfg_qDotMax"
  qDotAlgorithmMax/1 -> Apply Safety and Saturation/12(cfg_qDotAlgorithmMax)  "cfg_qDotAlgorithmMax"
  qMin/1 -> Apply Safety and Saturation/13(cfg_qMin)  "cfg_qMin"
  qMax/1 -> Apply Safety and Saturation/14(cfg_qMax)  "cfg_qMax"
  qLimitSoftMargin/1 -> Apply Safety and Saturation/15(cfg_qLimitSoftMargin)  "cfg_qLimitSoftMargin"
  cartesianLinearSpeedMax/1 -> Apply Safety and Saturation/16(cfg_cartesianLinearSpeedMax)  "cfg_cartesianLinearSpeedMax"
  focalRateGuaranteedMmPerSec/1 -> Apply Safety and Saturation/17(cfg_focalRateGuaranteedMmPerSec)  "cfg_focalRateGuaranteedMmPerSec"
  focalRateAbsoluteMaxMmPerSec/1 -> Apply Safety and Saturation/18(cfg_focalRateAbsoluteMaxMmPerSec)  "cfg_focalRateAbsoluteMaxMmPerSec"
  focalLengthWorkingMinMm/1 -> Apply Safety and Saturation/19(cfg_focalLengthWorkingMinMm)  "cfg_focalLengthWorkingMinMm"
  focalLengthWorkingMaxMm/1 -> Apply Safety and Saturation/20(cfg_focalLengthWorkingMaxMm)  "cfg_focalLengthWorkingMaxMm"
  focalLengthHardwareMinMm/1 -> Apply Safety and Saturation/21(cfg_focalLengthHardwareMinMm)  "cfg_focalLengthHardwareMinMm"
  focalLengthHardwareMaxMm/1 -> Apply Safety and Saturation/22(cfg_focalLengthHardwareMaxMm)  "cfg_focalLengthHardwareMaxMm"
  Ts/1 -> Apply Safety and Saturation/23(cfg_Ts)  "cfg_Ts"
  numericalEpsilon/1 -> Apply Safety and Saturation/24(cfg_numericalEpsilon)  "cfg_numericalEpsilon"
  armControlCalibrationReady/1 -> Apply Safety and Saturation/25(cfg_armControlCalibrationReady)  "cfg_armControlCalibrationReady"
  zoomControlCalibrationReady/1 -> Apply Safety and Saturation/26(cfg_zoomControlCalibrationReady)  "cfg_zoomControlCalibrationReady"
  armControlEnable/1 -> Apply Safety and Saturation/27(cfg_armControlEnable)  "cfg_armControlEnable"
  zoomControlEnable/1 -> Apply Safety and Saturation/28(cfg_zoomControlEnable)  "cfg_zoomControlEnable"
  Apply Safety and Saturation/1(qDotApplied) -> qDotApplied/1  "qDotApplied"
  Apply Safety and Saturation/2(fDotMmApplied) -> fDotMmApplied/1  "fDotMmApplied"
  Apply Safety and Saturation/3(qSaturationFlag) -> qSaturationFlag/1  "qSaturationFlag"
  Apply Safety and Saturation/4(focalRateSaturationFlag) -> focalRateSaturationFlag/1  "focalRateSaturationFlag"
  Apply Safety and Saturation/5(jointVelocitySaturationFlag) -> jointVelocitySaturationFlag/1  "jointVelocitySaturationFlag"
  Apply Safety and Saturation/6(jointVelocitySaturationAny) -> jointVelocitySaturationAny/1  "jointVelocitySaturationAny"
  Apply Safety and Saturation/7(jointLimitWarning) -> jointLimitWarning/1  "jointLimitWarning"
  Apply Safety and Saturation/8(cartesianSpeed) -> cartesianSpeed/1  "cartesianSpeed"
  Apply Safety and Saturation/9(cartesianSpeedScale) -> cartesianSpeedScale/1  "cartesianSpeedScale"
  Apply Safety and Saturation/10(cartesianSpeedSaturationFlag) -> cartesianSpeedSaturationFlag/1  "cartesianSpeedSaturationFlag"
  Apply Safety and Saturation/11(focalLengthCommandMm) -> focalLengthCommandMm/1  "focalLengthCommandMm"
  Apply Safety and Saturation/12(focalRateUsageGuaranteed) -> focalRateUsageGuaranteed/1  "focalRateUsageGuaranteed"
  Apply Safety and Saturation/13(focalRateUsageHard) -> focalRateUsageHard/1  "focalRateUsageHard"
  Apply Safety and Saturation/14(focalRateHardViolation) -> focalRateHardViolation/1  "focalRateHardViolation"
  Apply Safety and Saturation/15(safetyValid) -> safetyValid/1  "safetyValid"

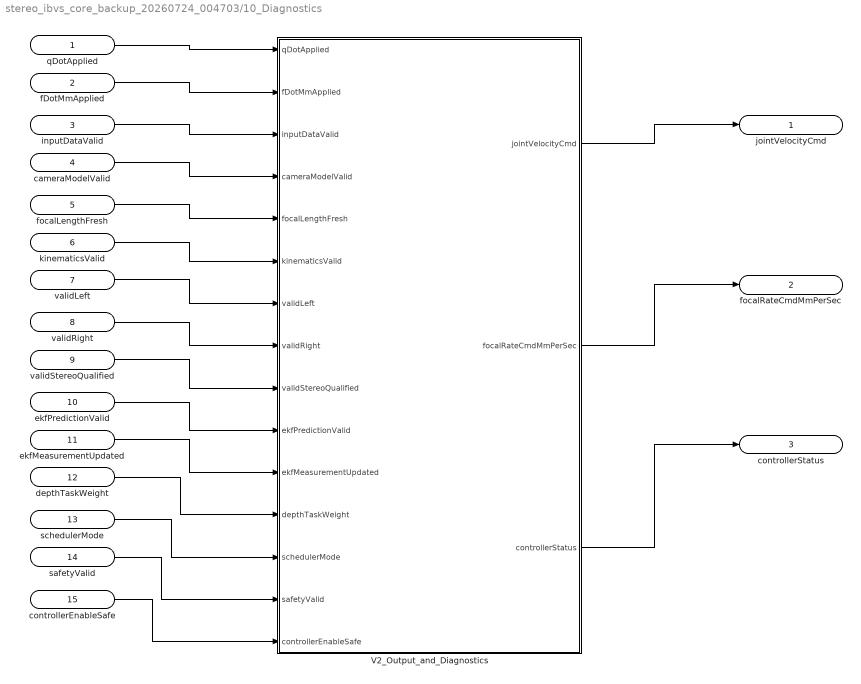
== system stereo_ibvs_core_backup_20260724_004703/10_Diagnostics ==
  qDotApplied : Inport  PortDimensions=7
  fDotMmApplied : Inport  Port=2  PortDimensions=2
  inputDataValid : Inport  Port=3  PortDimensions=1
  cameraModelValid : Inport  Port=4  PortDimensions=1
  focalLengthFresh : Inport  Port=5  PortDimensions=1
  kinematicsValid : Inport  Port=6  PortDimensions=1
  validLeft : Inport  Port=7  PortDimensions=1
  validRight : Inport  Port=8  PortDimensions=1
  validStereoQualified : Inport  Port=9  PortDimensions=1
  ekfPredictionValid : Inport  Port=10  PortDimensions=1
  ekfMeasurementUpdated : Inport  Port=11  PortDimensions=1
  depthTaskWeight : Inport  Port=12  PortDimensions=1
  schedulerMode : Inport  Port=13  PortDimensions=1
  safetyValid : Inport  Port=14  PortDimensions=1
  controllerEnableSafe : Inport  Port=15  PortDimensions=1
  V2_Output_and_Diagnostics : MATLAB Function  TreatAsAtomicUnit=on
  jointVelocityCmd : Outport  PortDimensions=7
  focalRateCmdMmPerSec : Outport  Port=2  PortDimensions=2
  controllerStatus : Outport  Port=3  PortDimensions=13
  wires:
  qDotApplied/1 -> V2_Output_and_Diagnostics/1(qDotApplied)
  fDotMmApplied/1 -> V2_Output_and_Diagnostics/2(fDotMmApplied)
  inputDataValid/1 -> V2_Output_and_Diagnostics/3(inputDataValid)
  cameraModelValid/1 -> V2_Output_and_Diagnostics/4(cameraModelValid)
  focalLengthFresh/1 -> V2_Output_and_Diagnostics/5(focalLengthFresh)
  kinematicsValid/1 -> V2_Output_and_Diagnostics/6(kinematicsValid)
  validLeft/1 -> V2_Output_and_Diagnostics/7(validLeft)
  validRight/1 -> V2_Output_and_Diagnostics/8(validRight)
  validStereoQualified/1 -> V2_Output_and_Diagnostics/9(validStereoQualified)
  ekfPredictionValid/1 -> V2_Output_and_Diagnostics/10(ekfPredictionValid)
  ekfMeasurementUpdated/1 -> V2_Output_and_Diagnostics/11(ekfMeasurementUpdated)
  depthTaskWeight/1 -> V2_Output_and_Diagnostics/12(depthTaskWeight)
  schedulerMode/1 -> V2_Output_and_Diagnostics/13(schedulerMode)
  safetyValid/1 -> V2_Output_and_Diagnostics/14(safetyValid)
  controllerEnableSafe/1 -> V2_Output_and_Diagnostics/15(controllerEnableSafe)
  V2_Output_and_Diagnostics/1(jointVelocityCmd) -> jointVelocityCmd/1
  V2_Output_and_Diagnostics/2(focalRateCmdMmPerSec) -> focalRateCmdMmPerSec/1
  V2_Output_and_Diagnostics/3(controllerStatus) -> controllerStatus/1
